simulink model "Receiver_UnderTest_Fixed"  (R2017b)
settings: Solver=FixedStepDiscrete  StartTime=0.0  StopTime=0.056214  RelTol=1e-3
InitFcn:
  | barker = comm.BarkerCode('SamplesPerFrame', 28, 'Length', 11);
  | seq = barker()+1;
  | M = 4;
  | hPSKModTrain   = comm.PSKModulator(M, ...
  |     'PhaseOffset',pi/4, ...
  |     'SymbolMapping','Binary');
  | xPreambleSeq = hPSKModTrain(seq);
  | 
  | 
  | %%%%%%%%%%%%
  | 
  | % AGC Preamble
  | reps = 5;
  | barker = comm.BarkerCode('SamplesPerFrame', 16, 'Length', 13);
  | seq = barker()+1;
  | %preamble = zeros(16*reps,1);
  | preambleFull = repmat(seq,reps,1);
  | rctFilt = comm.RaisedCosineTransmitFilter('FilterSpanInSymbols', 128,...
  | 'RolloffFactor',0.5,...
  | 'OutputSamplesPerSymbol',4);
  | preambleFullFilt = rctFilt(preambleFull);
  | 
  | %%%%%%%%%%%%
  | 
  | RadioSampleRate = 1e6;
  | %RadioSampleRate = 20e6;
  | RadioFrameLength = 1e5;
  | 
  | VibertiTracebackLength = 34+0;
  | numTrainingSamples = 250;
  | crc32Poly = [1 0 0 0 0 0 1 0 0 1 1 0 0 0 0 0 1 0 0 0 1 1 1 0 1 1 0 1 1 0 1 1 1];
  | crcDecodeLag = length(crc32Poly)-1+2;
  | 
  | %%%%%%%%%%%%
  | 
  | beta = 0.5;
  | span = 8;
  | sps = 4;
  | filterGain = 1;
  | coeff = rcosdesign(beta, span, sps, 'sqrt')*filterGain;
  | 
  | %%%%%%%%%%%%
  | 
  | samplesPerSymbol = 4;
  | maxPacketBits = 8*1500;
  | bItsPerSymbol = 2;
  | CodeRate = 2;
  | tailSymbols = 40;
  | maxPayloadSymbols = maxPacketBits*CodeRate/bItsPerSymbol+tailSymbols;
  | 
  | %%%%%%%%%%%%
  | 
  | NormalizedLoopBandwidths = 0.01:0.01:1;
  | K1 = zeros(length(NormalizedLoopBandwidths),1);
  | K2 = zeros(length(NormalizedLoopBandwidths),1);
  | 
  | for index=1:length(NormalizedLoopBandwidths)
  |     DampingFactor = 4*1/sqrt(2);
  |     samplesPerSymbols = 1;
  |     NormalizedLoopBandwidth = NormalizedLoopBandwidths(index);
  | 
  |     %%
  |     PhaseRecoveryLoopBandwidth = NormalizedLoopBandwidth*samplesPerSymbols;
  | 
  |     PhaseRecoveryGain = samplesPerSymbols;
  | 
  |     PhaseErrorDetectorGain = 1;
  | 
  |     %%
  |     theta = PhaseRecoveryLoopBandwidth/...
  |         ((DampingFactor + 0.25/DampingFactor)*samplesPerSymbols);
  | 
  |     d = 1 + 2*DampingFactor*theta + theta*theta;
  | 
  |     % K1
  |     K1(index) = (4*DampingFactor*theta/d)/...
  |         (PhaseErrorDetectorGain*PhaseRecoveryGain);
  |     % K2
  |     K2(index) = (4/samplesPerSymbols*theta*theta/d)/...
  |         (PhaseErrorDetectorGain*PhaseRecoveryGain);
  | 
  | end
  | K1 = fi(K1,0);
  | K2 = fi(K2,0);
libraries: commsource2 x1, RxTxFixedPointLibrary x1
settings Model: DataTypeOverride=Off  MinMaxOverflowLogging=MinMaxAndOverflow  FPTRunName=NoOverride  Creator=tcollins  LastModifiedBy=tcollins
settings DataIOCC: SaveFormat=Array  SaveOutput=off  SaveTime=off
settings OptimizationCC: BlockReduction=off  ConditionallyExecuteInputs=off  DefaultParameterBehavior=Inlined
settings DebuggingCC: AlgebraicLoopMsg=error  SingleTaskRateTransMsg=error
settings HardwareCC: ProdBitPerPointer=32  ProdBitPerSizeT=32  ProdBitPerPtrDiffT=32  ProdLargestAtomicFloat=None  ProdIntDivRoundTo=Undefined  ProdEndianess=Unspecified  ProdWordSize=32  ProdHWDeviceType=ASIC/FPGA->ASIC/FPGA  ProdEqTarget=off
settings CodeAppCC: StateflowObjectComments=on
settings SimscapeCC: SimscapeNormalizeSystem=off

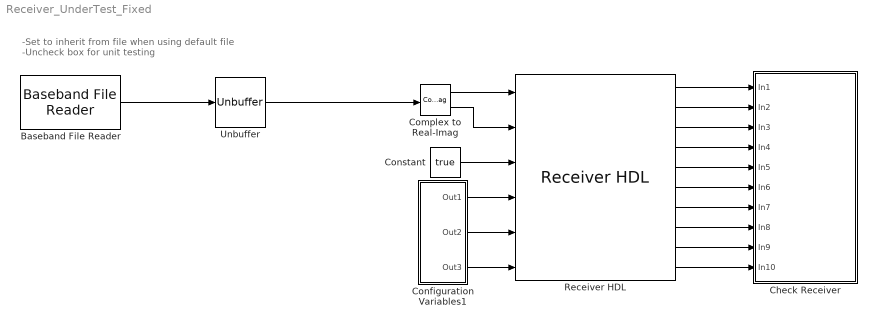
== system Receiver_UnderTest_Fixed ==
  note: -Set to inherit from file when using default file
      | -Uncheck box for unit testing
  Baseband File Reader : commsource2/Baseband File Reader  Filename=PlutoCaptureQPSK.bb  InheritSampleTimeFromFile=off  SampleTime=100000/RadioSampleRate  SamplesPerFrame=100000  CyclicRepetition=off  FileEndOutputPort=off  SimulateUsing=Interpreted execution
      settings: SourceProductName=Communications System Toolbox  SourceProductBaseCode=CM
  Check Receiver : Subsystem
  Complex to Real-Imag : ComplexToRealImag
  Configuration Variables1 : Subsystem
  Constant : Constant  Value=true  SampleTime=1/RadioSampleRate
  Receiver HDL : RxTxFixedPointLibrary/Receiver HDL  SystemSampleTime=-1
  Unbuffer : Unbuffer
  wires:
  Constant/1 -> Receiver HDL/3
  Complex to Real-Imag/2 -> Receiver HDL/2
  Baseband File Reader/1 -> Unbuffer/1
  Unbuffer/1 -> Complex to Real-Imag/1
  Configuration Variables1/1(Out1) -> Receiver HDL/4
  Configuration Variables1/2(Out2) -> Receiver HDL/5
  Configuration Variables1/3(Out3) -> Receiver HDL/6
  Complex to Real-Imag/1 -> Receiver HDL/1
  Receiver HDL/1 -> Check Receiver/1(In1)
  Receiver HDL/2 -> Check Receiver/2(In2)
  Receiver HDL/3 -> Check Receiver/3(In3)
  Receiver HDL/4 -> Check Receiver/4(In4)
  Receiver HDL/5 -> Check Receiver/5(In5)
  Receiver HDL/6 -> Check Receiver/6(In6)
  Receiver HDL/7 -> Check Receiver/7(In7)
  Receiver HDL/8 -> Check Receiver/8(In8)
  Receiver HDL/9 -> Check Receiver/9(In9)
  Receiver HDL/10 -> Check Receiver/10(In10)

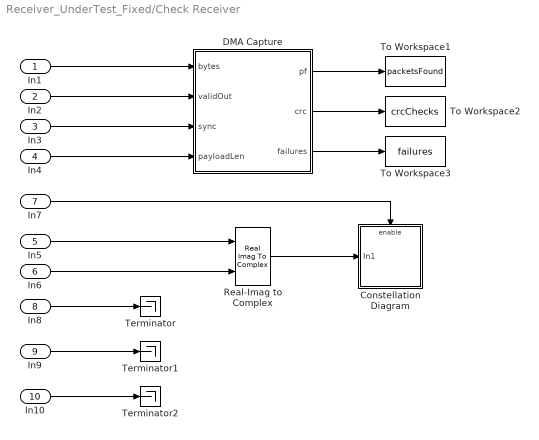
== system Receiver_UnderTest_Fixed/Check Receiver ==
  In1 : Inport
  In2 : Inport  Port=2
  In3 : Inport  Port=3
  In4 : Inport  Port=4
  In5 : Inport  Port=5
  In6 : Inport  Port=6
  In7 : Inport  Port=7
  In8 : Inport  Port=8
  In9 : Inport  Port=9
  In10 : Inport  Port=10
  Constellation Diagram : Subsystem
  DMA Capture : MATLAB Function  TreatAsAtomicUnit=on
  Real-Imag to Complex : RealImagToComplex
  Terminator : Terminator
  Terminator1 : Terminator
  Terminator2 : Terminator
  To Workspace1 : ToWorkspace  VariableName=packetsFound  SaveFormat=Timeseries  SampleTime=-1
  To Workspace2 : ToWorkspace  VariableName=crcChecks  SaveFormat=Timeseries  SampleTime=-1
  To Workspace3 : ToWorkspace  VariableName=failures  SaveFormat=Timeseries  SampleTime=-1
  wires:
  Real-Imag to Complex/1 -> Constellation Diagram/1(In1)
  In5/1 -> Real-Imag to Complex/1
  In3/1 -> DMA Capture/3(sync)
  In7/1 -> Constellation Diagram/Enable
  In2/1 -> DMA Capture/2(validOut)
  In1/1 -> DMA Capture/1(bytes)
  In4/1 -> DMA Capture/4(payloadLen)
  In6/1 -> Real-Imag to Complex/2
  DMA Capture/1(pf) -> To Workspace1/1
  DMA Capture/2(crc) -> To Workspace2/1
  DMA Capture/3(failures) -> To Workspace3/1
  In8/1 -> Terminator/1
  In9/1 -> Terminator1/1
  In10/1 -> Terminator2/1

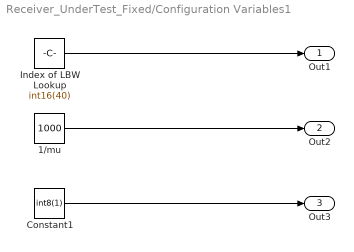
== system Receiver_UnderTest_Fixed/Configuration Variables1 ==
  1/mu : Constant  Value=1000  OutDataTypeStr=int16  SampleTime=-1
  Constant1 : Constant  Value=int8(1)  SampleTime=1/RadioSampleRate
  Index of LBW Lookup : Constant  Value=int16(40)  SampleTime=1/RadioSampleRate
  Out1 : Outport
  Out2 : Outport  Port=2
  Out3 : Outport  Port=3
  wires:
  1/mu/1 -> Out2/1
  Index of LBW Lookup/1 -> Out1/1
  Constant1/1 -> Out3/1

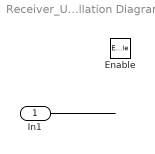
== system Receiver_UnderTest_Fixed/Check Receiver/Constellation Diagram ==
  In1 : Inport
  Enable : EnablePort
  wires:
  In1/1 -> ?

== matlab function Receiver_UnderTest_Fixed/Check Receiver/DMA Capture ==
  data: bytes input; validOut input; sync input; payloadLen input; pf output; crc output; failures output
function [pf, crc, failures] = fcn(bytes, validOut, sync, payloadLen)

persistent frameBuffer byteCounter fullPayloadBits result

bitsInPack = 64;

if isempty(frameBuffer)
    maxFrameBits = (2^16)*8;
    frameBuffer = false(maxFrameBits,1);
    byteCounter = 0;
    fullPayloadBits = uint16(0);
    result = struct('packetsFound',0,...
    'crcChecks',zeros(1,100),'failures',zeros(1,100));
end

if validOut
    if sync
        byteCounter = bitsInPack;
        frameBuffer(1:byteCounter) = bitget(bytes,1:bitsInPack);
        fullPayloadBits = uint16(payloadLen*8);
        
    elseif byteCounter<fullPayloadBits
        frameBuffer(byteCounter+1:byteCounter+bitsInPack) = bitget(bytes,1:bitsInPack);
        byteCounter = byteCounter + bitsInPack;
    else
        result.packetsFound = result.packetsFound + 1;
        if bytes>0
            fprintf('CRC Error (Exterior Check) [Len: %u]\n',fullPayloadBits);
            result.crcChecks(result.packetsFound) = 1;
            result.failures(result.packetsFound) = 4;
        else
            fprintf('Frame passed CRC (Exterior Check) [Len: %u]\n',fullPayloadBits);
        end
    end
end

pf = result.packetsFound;
crc = result.crcChecks;
failures = result.failures;
